simulink model "lab1_traffic_lights"  (R2023b)
settings: Solver=FixedStepAuto  StartTime=0.0  StopTime=10.0  RelTol=1e-3  EnableMultiTasking=on
libraries: arduinolib x3
settings Model: ExtModeTrigDuration=2  Creator=ascom  LastModifiedBy=ascom
settings OptimizationCC: EnhancedBackFolding=on  PassReuseOutputArgsAs=Individual arguments  ZeroExternalMemoryAtStartup=off  ZeroInternalMemoryAtStartup=off  MaxStackSize=64  OptimizeBlockOrder=speed  DifferentSizesBufferReuse=on  OptimizationCustomize=off  EfficientTunableParamExpr=on
settings DebuggingCC: ParameterTunabilityLossMsg=error
settings HardwareCC: ProdBitPerInt=16  ProdBitPerPointer=16  ProdBitPerSizeT=16  ProdBitPerPtrDiffT=16  ProdLargestAtomicFloat=None  ProdWordSize=8  ProdHWDeviceType=Atmel->AVR
settings SFSimCC: MATLABDynamicMemAlloc=off
settings RTWCC: Description=Embedded Coder  SystemTargetFile=ert.tlc  HardwareBoard=Arduino Uno  TemplateMakefile=ert_default_tmf  Toolchain=Arduino AVR  BuildConfiguration=Faster Runs
settings CodeAppCC: ForceParamTrailComments=on  IgnoreCustomStorageClasses=off  OperatorAnnotations=on  SimulinkDataObjDesc=on  SFDataObjDesc=on  InsertBlockDesc=on
settings ERTTargetCC: SupportContinuousTime=on  SupportVariableSizeSignals=on  ExtModeTransport=3  ExtModeStaticAlloc=on  ExtModeAutomaticAllocSize=off  ExtModeStaticAllocSize=250  ExtModeMexFile=ext_xcp  ExtModeIntrfLevel=Level2 - Open

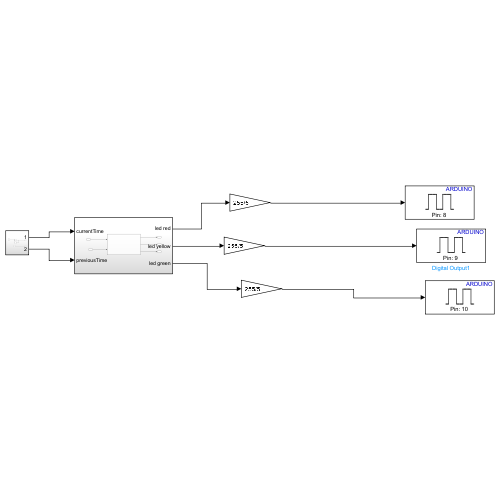
[thumbnail: Simulink's stored preview of the top-level diagram]
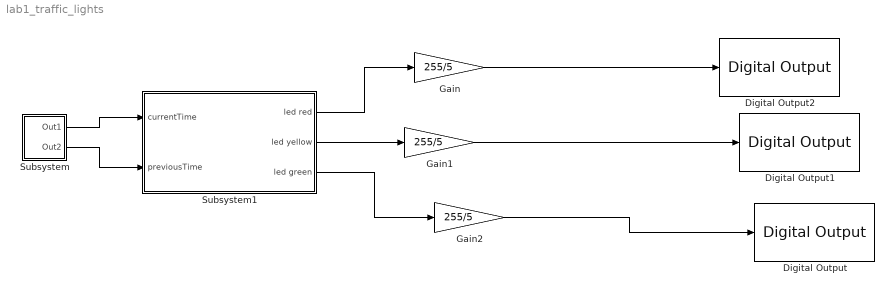
== system lab1_traffic_lights ==
  Digital Output : arduinolib/Digital Output  pinNumber=10  Direction=output  blockPlatform=arduino
  Digital Output1 : arduinolib/Digital Output  pinNumber=9  Direction=output  blockPlatform=arduino
  Digital Output2 : arduinolib/Digital Output  pinNumber=8  Direction=output  blockPlatform=arduino
  Gain : Gain  Gain=255/5
  Gain1 : Gain  Gain=255/5
  Gain2 : Gain  Gain=255/5
  Subsystem : Subsystem
  Subsystem1 : Subsystem
  wires:
  Subsystem/1(Out1) -> Subsystem1/1(currentTime)
  Subsystem/2(Out2) -> Subsystem1/2(previousTime)
  Subsystem1/1(led red) -> Gain/1
  Subsystem1/2(led yellow) -> Gain1/1
  Subsystem1/3(led green) -> Gain2/1
  Gain/1 -> Digital Output2/1
  Gain1/1 -> Digital Output1/1
  Gain2/1 -> Digital Output/1

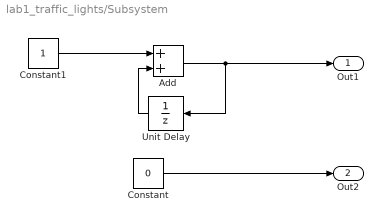
== system lab1_traffic_lights/Subsystem ==
  Add : Sum
  Constant : Constant  Value=0
  Constant1 : Constant
  Unit Delay : UnitDelay  SampleTime=2  HasFrameUpgradeWarning=on
  Out1 : Outport
  Out2 : Outport  Port=2
  wires:
  Unit Delay/1 -> Add/2
  Add/1 -> Out1/1, Unit Delay/1
  Constant/1 -> Out2/1
  Constant1/1 -> Add/1

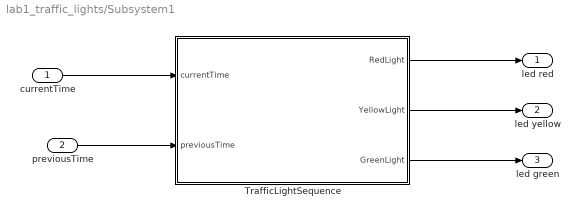
== system lab1_traffic_lights/Subsystem1 ==
  currentTime : Inport
  previousTime : Inport  Port=2
  TrafficLightSequence : MATLAB Function  TreatAsAtomicUnit=on
  led red : Outport
  led yellow : Outport  Port=2
  led green : Outport  Port=3
  wires:
  TrafficLightSequence/3(GreenLight) -> led green/1
  TrafficLightSequence/2(YellowLight) -> led yellow/1
  TrafficLightSequence/1(RedLight) -> led red/1
  currentTime/1 -> TrafficLightSequence/1(currentTime)
  previousTime/1 -> TrafficLightSequence/2(previousTime)

== matlab function lab1_traffic_lights/Subsystem1/TrafficLightSequence ==
  data: currentTime input; RedLight output; previousTime input; YellowLight output; GreenLight output
function [RedLight, YellowLight, GreenLight] = TrafficLightSequenceContinuous(currentTime, previousTime)
    % Continuous traffic light sequence
    
    % Adjust timing parameters (in seconds)
    redTime = 2;     % Set the duration for the red light
    yellowTime = 2;   % Set the duration for the yellow light
    greenTime = 2;   % Set the duration for the green light

    % Initialize outputs
    RedLight = 0;
    YellowLight = 0;
    GreenLight = 0;

    % Calculate elapsed time since the last update
    elapsedTime = currentTime - previousTime;

    % Calculate the time within a complete cycle
    cycleTime = redTime + yellowTime + greenTime;

    % Determine the current phase in the cycle
    currentPhase = mod(elapsedTime, cycleTime);

    % Traffic light sequence logic
    if currentPhase < redTime
        % Red light is ON
        RedLight = 1;
    elseif currentPhase < redTime + yellowTime
        % Yellow light is ON
        YellowLight = 1;
    else
        % Green light is ON
        GreenLight = 1;
    end
end
